simulink model "chapter12"  (R2021b)
settings: Solver=FixedStepAuto  StartTime=0.0  StopTime=50  FixedStep=0.001  RelTol=1e-3
model workspace (MAT data in the model file):
  Np = 1
libraries: slpidlib x1, simulink x1
settings Model: Creator=Mohammad  LastModifiedBy=Saeed Bab
settings SolverCC: AlgebraicLoopSolver=TrustRegion
settings DebuggingCC: SFMachineParentedDataDiag=warning

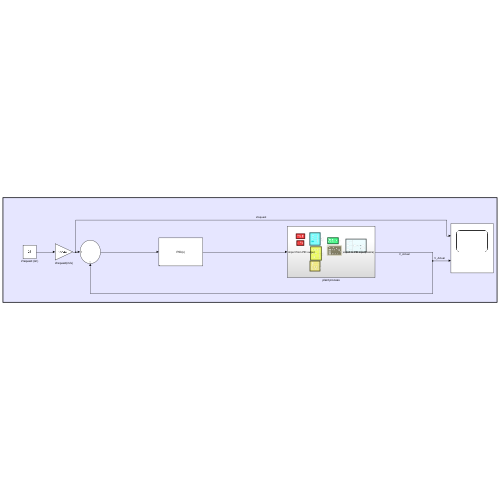
[thumbnail: Simulink's stored preview of the top-level diagram]
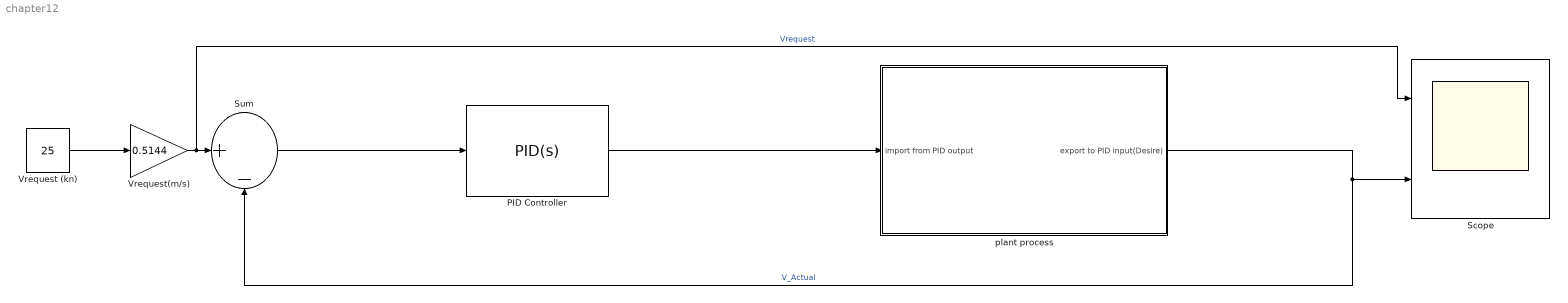
== system chapter12 ==
  PID Controller : slpidlib/PID Controller  Controller=PID  Form=Parallel  TimeDomain=Continuous-time  UseExternalTs=off  SampleTime=-1  IntegratorMethod=Forward Euler  FilterMethod=Forward Euler  ControllerParametersSource=internal  P=5  I=2  D=0  UseFilter=on  N=100  TunerSelectOption=Transfer Function Based (PID Tuner App)  InitialConditionSource=internal  InitialConditionForIntegrator=0  InitialConditionForFilter=0  DifferentiatorICPrevScaledInput=0  ExternalReset=none  TrackingMode=off  Kt=1  LimitOutput=off  SatLimitsSource=internal  UpperSaturationLimit=inf  LowerSaturationLimit=-inf  LinearizeAsGain=on  AntiWindupMode=none  Kb=1  POutMin=[]  POutMax=[]  IOutMin=[]  IOutMax=[]  DOutMin=[]  DOutMax=[]  NOutMin=[]  NOutMax=[]  SumOutMin=[]  SumOutMax=[]  SaturationOutMin=[]  SaturationOutMax=[]  PParamMin=[]  PParamMax=[]  IParamMin=[]  IParamMax=[]  DParamMin=[]  DParamMax=[]  NParamMin=[]  NParamMax=[]  KbParamMin=[]  KbParamMax=[]  KtParamMin=[]  KtParamMax=[]  KbOutMin=[]  KbOutMax=[]  KtOutMin=[]  KtOutMax=[]  IntegratorOutMin=[]  IntegratorOutMax=[]  FilterOutMin=[]  FilterOutMax=[]  SumI1OutMin=[]  SumI1OutMax=[]  SumI2OutMin=[]  SumI2OutMax=[]  SumI3OutMin=[]  SumI3OutMax=[]  SumI4OutMin=[]  SumI4OutMax=[]  SumDOutMin=[]  SumDOutMax=[]  DifferentiatorOutMin=[]  DifferentiatorOutMax=[]  FilterDiffOutCoefMin=[]  FilterDiffOutCoefMax=[]  ReciprocalOutMin=[]  ReciprocalOutMax=[]  SumDenOutMin=[]  SumDenOutMax=[]  SumNumOutMin=[]  SumNumOutMax=[]  DivideOutMin=[]  DivideOutMax=[]  UdiffTsProdOutMin=[]  UdiffTsProdOutMax=[]  NTsProdOutMin=[]  NTsProdOutMax=[]  UintegralTsProdOutMin=[]  UintegralTsProdOutMax=[]  UngainTsProdOutMin=[]  UngainTsProdOutMax=[]  IntegratorContinuousStateAttributes=''  IntegratorStateMustResolveToSignalObject=off  IntegratorRTWStateStorageClass=Auto  FilterContinuousStateAttributes=''  FilterStateMustResolveToSignalObject=off  FilterRTWStateStorageClass=Auto  ParallelPVariant=InternalParameters  IdealPVariant=Disabled  IVariant=InternalParameters  DVariant=InternalParameters  IntegratorVariant=Continuous  SatVariant=Disabled  AWVariant=Passthrough  PCopyVariant=Disabled  TRVariant=Disabled  FdbkBlocksVariant=Forward  IdealPFdbkVariant=Disabled  SatFdbkVariant=Disabled  DerivativeFilterVariant=ContFilter  NVariant=InternalParameters  NCopyVariant=Disabled  FilterICVariant=InternalICsFilter  IntegratorICVariant=InternalICs  ExternalResetVariant=Disabled  TRSumVariant=Passthrough  SumFdbkVariant=Disabled  SumVariant=Sum_PID  TsampFilterVariant=InternalTs  TsampNgainVariant=Passthrough  TsampIntegralVariant=Passthrough  ExternalSaturationOutDataTypeStr=Inherit: Same as second input
  Scope : Scope  NumInputPorts=2
  Sum : Sum  Inputs=|+-
  Vrequest (kn) : Constant  Value=25
  Vrequest(m/s) : Gain  Gain=0.5144
  plant process : Subsystem
  wires:
  Vrequest (kn)/1 -> Vrequest(m/s)/1
  Vrequest(m/s)/1 -> Sum/1, Scope/1  "Vrequest"
  plant process/1(export to PID input(Desire)) -> Sum/2, Scope/2  "V_Actual"
  Sum/1 -> PID Controller/1
  PID Controller/1 -> plant process/1(import from PID output)

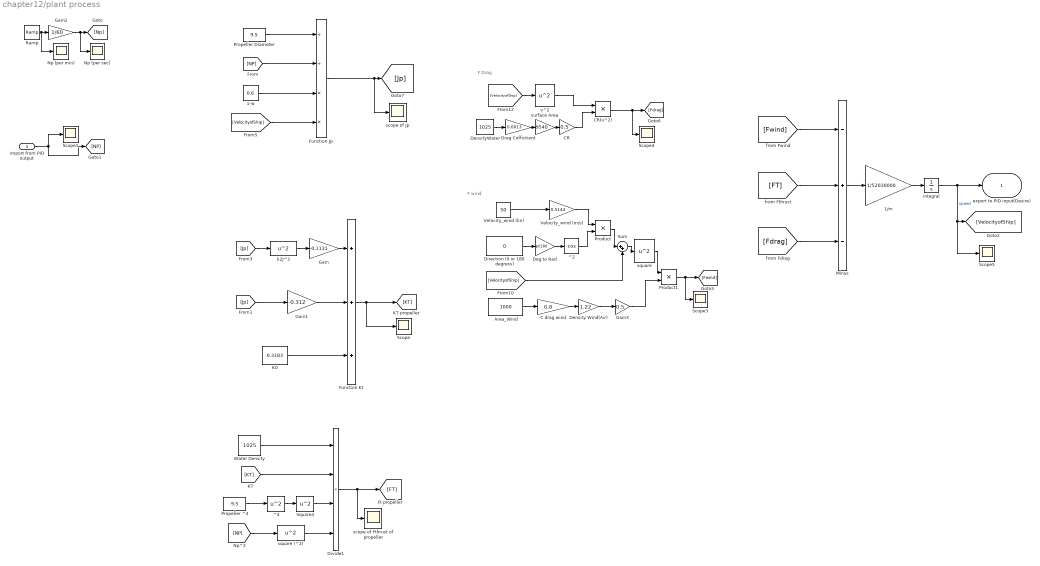
== system chapter12/plant process ==
  note: F Drag
  note: F wind
  import from PID output : Inport
  " Direction (0 or 180 degress)" : Constant  Value=0
  " ^4" : Math  Operator=square  SaturateOnIntegerOverflow=on
  1-w : Constant  Value=0.6
  1/m : Gain  Gain=1/52030000
  Area_Wind : Constant  Value=1000
  C drag wind : Gain  Gain=0.8
  CR : Gain  Gain=0.5
  CR(u^2) : Product
  Deg to Rad : Gain  Gain=pi/180
  Density Wind(Air) : Gain  Gain=1.22
  "DensityWater " : Constant  Value=1025
  Divide1 : Product  Inputs=****
  Drag Coffictient : Gain  Gain=0.0013
  Function Jp : Product  Inputs=//**
  Function Kt : Sum  Inputs=+++
  Gain : Gain  Gain=-0.1131
  Gain1 : Gain  Gain=-0.312
  Gain2 : Gain  Gain=1/60
  Gain3 : Gain  Gain=0.5
  K0 : Constant  Value=0.3183
  Minus : Sum  Inputs=-+-
  Np (per min) : Scope
  Np (per sec) : Scope
  Product : Product
  Product1 : Product
  Propeller Diameter : Constant  Value=9.5
  Propeller ^4 : Constant  Value=9.5
  Ramp : simulink/Sources/Ramp  slope=0.75  start=0  InitialOutput=0.01
  Scope{,1,3..5} (5 alike) : Scope
  Square4 : Math  Operator=square  SaturateOnIntegerOverflow=on
  Sum : Sum  Inputs=|++
  Velocity_wind (kn) : Constant  Value=50
  Velocity_wind (m/s) : Gain  Gain=0.5144
  Water Density : Constant  Value=1025
  ^2 : Trigonometry  Operator=cos  OutputSignalType=real
  integral : Integrator
  k2J^2 : Math  Operator=square  SaturateOnIntegerOverflow=on
  scope of Fthrust of propeller : Scope
  scope of Jp : Scope
  square : Math  Operator=square  SaturateOnIntegerOverflow=on
  square (^2) : Math  Operator=square  SaturateOnIntegerOverflow=on
  surface Area : Gain  Gain=9540
  v^2 : Math  Operator=square  SaturateOnIntegerOverflow=on
  export to PID input(Desire) : Outport
  wires:
  Deg to Rad/1 -> ^2/1
  " Direction (0 or 180 degress)"/1 -> Deg to Rad/1
  [VelocityofShip] -> v^2/1
  Velocity_wind (kn)/1 -> Velocity_wind (m/s)/1
  [NP] -> square (^2)/1
  Divide1/1 -> scope of Fthrust of propeller/1, [FT]
  v^2/1 -> CR(u^2)/1
  integral/1 -> [VelocityofShip], Scope5/1, export to PID input(Desire)/1  "speed"
  Minus/1 -> 1/m/1
  1/m/1 -> integral/1
  " ^4"/1 -> Square4/1
  Function Jp/1 -> scope of Jp/1, [Jp]
  Propeller Diameter/1 -> Function Jp/1
  [NP] -> Function Jp/2
  1-w/1 -> Function Jp/3
  [VelocityofShip] -> Function Jp/4
  Propeller ^4/1 -> " ^4"/1
  square (^2)/1 -> Divide1/4
  Square4/1 -> Divide1/3
  [KT] -> Divide1/2
  Water Density/1 -> Divide1/1
  Velocity_wind (m/s)/1 -> Product/1
  ^2/1 -> Product/2
  Product/1 -> Sum/1
  [VelocityofShip] -> Sum/2
  Sum/1 -> square/1
  Ramp/1 -> Np (per min)/1, Gain2/1
  Gain2/1 -> Np (per sec)/1, [Np]
  [Jp] -> k2J^2/1
  Gain1/1 -> Function Kt/2
  [Jp] -> Gain1/1
  K0/1 -> Function Kt/3
  k2J^2/1 -> Gain/1
  Function Kt/1 -> Scope/1, [KT]
  Gain/1 -> Function Kt/1
  "DensityWater "/1 -> Drag Coffictient/1
  Drag Coffictient/1 -> surface Area/1
  surface Area/1 -> CR/1
  CR/1 -> CR(u^2)/2
  CR(u^2)/1 -> Scope4/1, [Fdrag]
  Area_Wind/1 -> C drag wind/1
  C drag wind/1 -> Density Wind(Air)/1
  Gain3/1 -> Product1/2
  square/1 -> Product1/1
  Product1/1 -> Scope3/1, [Fwind]
  Density Wind(Air)/1 -> Gain3/1
  [FT] -> Minus/2
  [Fdrag] -> Minus/3
  [Fwind] -> Minus/1
  import from PID output/1 -> [NP], Scope1/1
